simulink model "BLDC"  (R2014b)
settings: Solver=ode45  StartTime=0.0  StopTime=.3  MaxStep=.0001  RelTol=1e-3
values from neighbouring files (symbols this model uses):
  A = [-r/l,0,0,0 ... (first row only)    [motorParams.m]
  B = [2/(3*l),1/(3*l),0 ... (first row only)    [motorParams.m]
  C = [1,0,0,0 ... (first row only)    [motorParams.m]
  c0 = .001    (= 0.001)    [motorParams.m]
  D = [0,0,0 ... (first row only)    [motorParams.m]
  encoderResolution = 12    [motorParams.m]
  encoderSampleTime = .001    (= 0.001)    [motorParams.m]
  ke = 1/(285*2*pi/60)    (= 0.0335063038088)    [motorParams.m]
  kt = 33.5e-3    (= 0.0335)    [motorParams.m]
  p = poles    (= 16)    [motorParams.m]

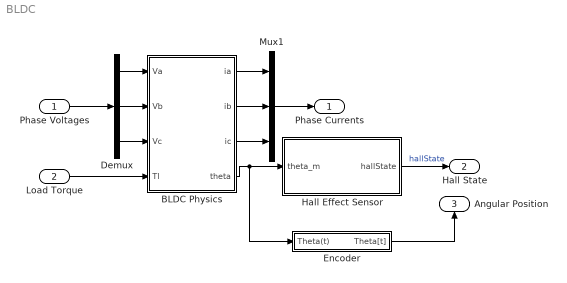
== system BLDC ==
  Phase Voltages : Inport  OutDataTypeStr=double  PortDimensions=3  SampleTime=0
  Load Torque : Inport  Port=2  OutDataTypeStr=double  PortDimensions=1  SampleTime=[0,0]
  BLDC Physics : Subsystem
  Demux : Demux  Outputs=3
  Encoder : Subsystem
  Hall Effect Sensor : MATLAB Function  TreatAsAtomicUnit=on
  Mux1 : Mux  Inputs=3
  Phase Currents : Outport  OutDataTypeStr=double  PortDimensions=3  SampleTime=0
  Hall State : Outport  Port=2  OutDataTypeStr=double  PortDimensions=[1 3]  SampleTime=0
  Angular Position : Outport  Port=3  OutDataTypeStr=double  PortDimensions=1  SampleTime=[0.001,0]
  wires:
  Hall Effect Sensor/1(hallState) -> Hall State/1  "hallState"
  Load Torque/1 -> BLDC Physics/4(Tl)
  BLDC Physics/4(theta) -> Hall Effect Sensor/1(theta_m), Encoder/1(Theta(t))
  Mux1/1 -> Phase Currents/1
  BLDC Physics/3(ic) -> Mux1/3
  BLDC Physics/2(ib) -> Mux1/2
  BLDC Physics/1(ia) -> Mux1/1
  Demux/3 -> BLDC Physics/3(Vc)
  Phase Voltages/1 -> Demux/1
  Demux/1 -> BLDC Physics/1(Va)
  Demux/2 -> BLDC Physics/2(Vb)
  Encoder/1("Theta[t] ") -> Angular Position/1

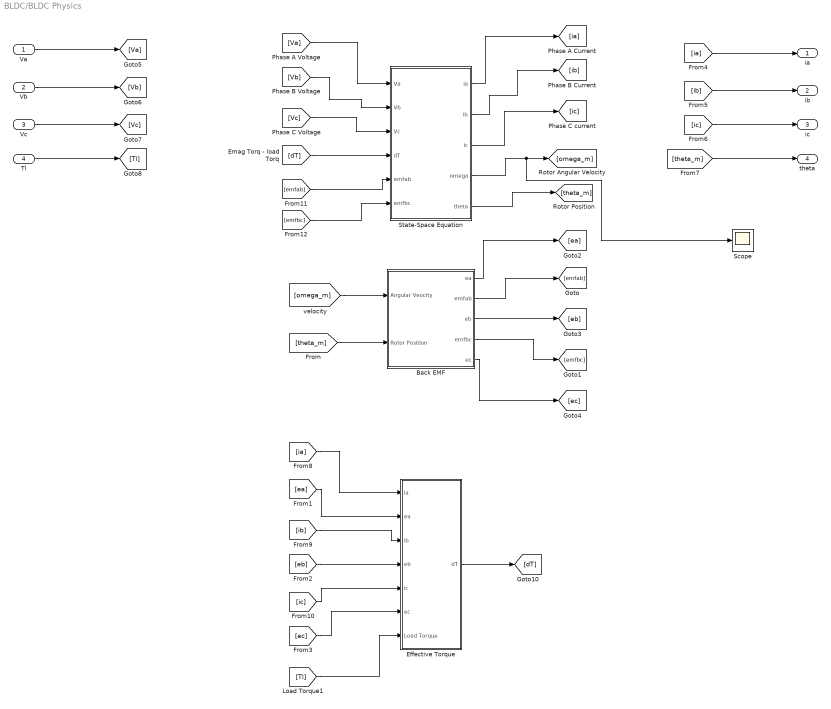
== system BLDC/BLDC Physics ==
  Va : Inport
  Vb : Inport  Port=2
  Vc : Inport  Port=3
  Tl : Inport  Port=4
  Back EMF : Subsystem
  Effective Torque : Subsystem
  Scope : Scope
  State-Space Equation : Subsystem
  ia : Outport
  ib : Outport  Port=2
  ic : Outport  Port=3
  theta : Outport  Port=4
  wires:
  [emfbc] -> State-Space Equation/6(emfbc)
  [emfab] -> State-Space Equation/5(emfab)
  Back EMF/4(emfbc) -> [emfbc]
  Vb/1 -> [Vb]
  Va/1 -> [Va]
  [theta_m] -> Back EMF/2(Rotor Position)
  Back EMF/1(ea) -> [ea]
  Tl/1 -> [Tl]
  [ia] -> ia/1
  [theta_m] -> theta/1
  Back EMF/3(eb) -> [eb]
  [ic] -> ic/1
  Vc/1 -> [Vc]
  [ib] -> ib/1
  Back EMF/5(ec) -> [ec]
  [omega_m] -> Back EMF/1(Angular Veocity)
  Back EMF/2(emfab) -> [emfab]
  [eb] -> Effective Torque/4(eb)
  [Tl] -> Effective Torque/7(Load Torque)
  [ic] -> Effective Torque/5(ic)
  [ea] -> Effective Torque/2(ea)
  [ia] -> Effective Torque/1(ia)
  [ec] -> Effective Torque/6(ec)
  [ib] -> Effective Torque/3(ib)
  Effective Torque/1(dT) -> [dT]
  [Vc] -> State-Space Equation/3(Vc)
  State-Space Equation/3(ic) -> [ic]
  State-Space Equation/4(omega) -> [omega_m], Scope/1
  [Vb] -> State-Space Equation/2(Vb)
  [dT] -> State-Space Equation/4(dT)
  State-Space Equation/2(ib) -> [ib]
  State-Space Equation/5(theta) -> [theta_m]
  [Va] -> State-Space Equation/1(Va)
  State-Space Equation/1(ia) -> [ia]

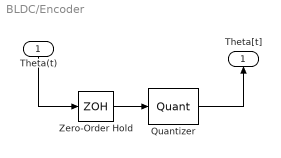
== system BLDC/Encoder ==
  Theta(t) : Inport
  Quantizer : Quantizer  QuantizationInterval=2*pi/(2^encoderResolution)
  Zero-Order Hold : ZeroOrderHold  SampleTime=encoderSampleTime
  "Theta[t] " : Outport
  wires:
  Zero-Order Hold/1 -> Quantizer/1
  Theta(t)/1 -> Zero-Order Hold/1
  Quantizer/1 -> "Theta[t] "/1

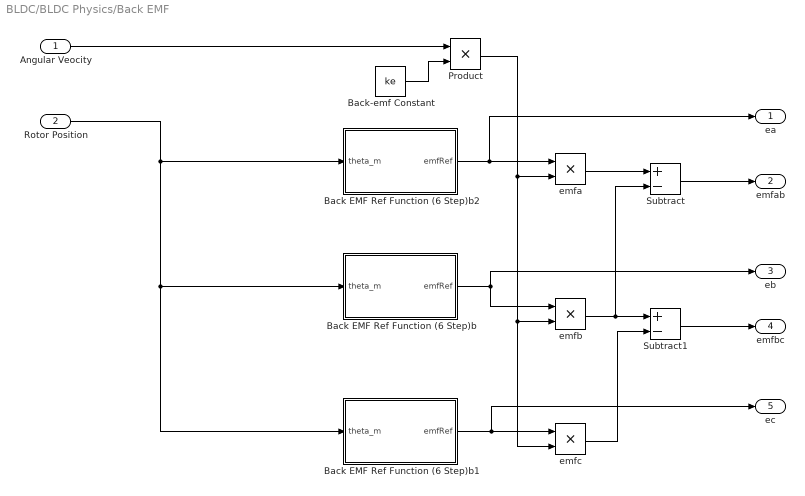
== system BLDC/BLDC Physics/Back EMF ==
  Angular Veocity : Inport
  Rotor Position : Inport  Port=2
  Back EMF Ref Function (6 Step)b : MATLAB Function  TreatAsAtomicUnit=on  mask{offset=-2*pi/3, p=p}
      mask prompts: offset "Phase shift"; p "Number of poles"
  Back EMF Ref Function (6 Step)b1 : MATLAB Function  TreatAsAtomicUnit=on  mask{offset=2*pi/3, p=p}
      mask prompts: offset "Phase shift"; p "Number of poles"
  Back EMF Ref Function (6 Step)b2 : MATLAB Function  TreatAsAtomicUnit=on  mask{offset=0, p=p}
      mask prompts: offset "Phase shift"; p "Number of poles"
  Back-emf Constant : Constant  Value=ke
  Product : Product
  Subtract : Sum  Inputs=+-
  Subtract1 : Sum  Inputs=+-
  emfa : Product
  emfb : Product
  emfc : Product
  ea : Outport
  emfab : Outport  Port=2
  eb : Outport  Port=3
  emfbc : Outport  Port=4
  ec : Outport  Port=5
  wires:
  Subtract1/1 -> emfbc/1
  Subtract/1 -> emfab/1
  emfa/1 -> Subtract/1
  Angular Veocity/1 -> Product/1
  Back EMF Ref Function (6 Step)b1/1(emfRef) -> emfc/1, ec/1
  Back EMF Ref Function (6 Step)b/1(emfRef) -> emfb/1, eb/1
  emfb/1 -> Subtract1/1, Subtract/2
  Product/1 -> emfb/2, emfc/2, emfa/2
  Back-emf Constant/1 -> Product/2
  emfc/1 -> Subtract1/2
  Back EMF Ref Function (6 Step)b2/1(emfRef) -> emfa/1, ea/1
  Rotor Position/1 -> Back EMF Ref Function (6 Step)b/1(theta_m), Back EMF Ref Function (6 Step)b1/1(theta_m), Back EMF Ref Function (6 Step)b2/1(theta_m)

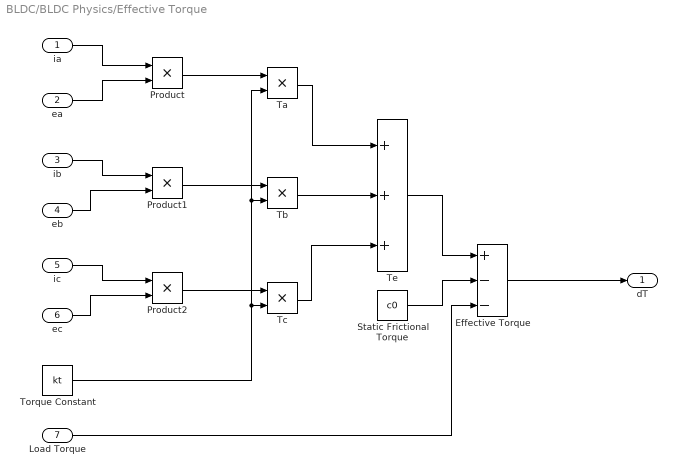
== system BLDC/BLDC Physics/Effective Torque ==
  ia : Inport
  ea : Inport  Port=2
  ib : Inport  Port=3
  eb : Inport  Port=4
  ic : Inport  Port=5
  ec : Inport  Port=6
  Load Torque : Inport  Port=7
  Effective Torque : Sum  Inputs=+--
  Product : Product
  Product1 : Product
  Product2 : Product
  Static Frictional Torque : Constant  Value=c0
  Ta : Product  Inputs=**
  Tb : Product  Inputs=**
  Tc : Product  Inputs=**
  Te : Sum  Inputs=+++
  Torque Constant : Constant  Value=kt
  dT : Outport
  wires:
  Te/1 -> Effective Torque/1
  Product2/1 -> Tc/1
  Product1/1 -> Tb/1
  Product/1 -> Ta/1
  Torque Constant/1 -> Ta/2, Tb/2, Tc/2
  Effective Torque/1 -> dT/1
  ia/1 -> Product/1
  ic/1 -> Product2/1
  ea/1 -> Product/2
  ib/1 -> Product1/1
  eb/1 -> Product1/2
  ec/1 -> Product2/2
  Tb/1 -> Te/2
  Ta/1 -> Te/1
  Tc/1 -> Te/3
  Load Torque/1 -> Effective Torque/3
  Static Frictional Torque/1 -> Effective Torque/2

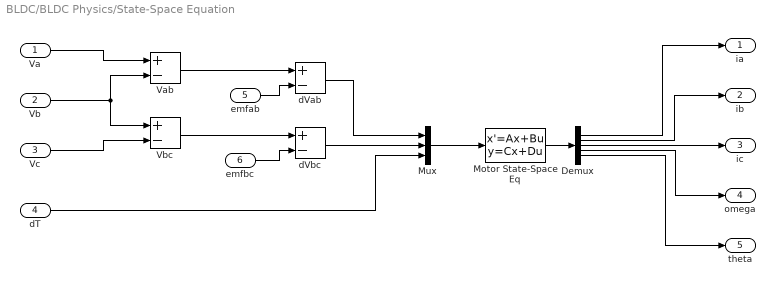
== system BLDC/BLDC Physics/State-Space Equation ==
  Va : Inport
  Vb : Inport  Port=2
  Vc : Inport  Port=3
  dT : Inport  Port=4
  emfab : Inport  Port=5
  emfbc : Inport  Port=6
  Demux : Demux  Outputs=5
  Motor State-Space Eq : StateSpace  A=A  B=B  C=C  D=D  X0=0
  Mux : Mux  Inputs=3
  Vab : Sum  Inputs=+-
  Vbc : Sum  Inputs=+-
  dVab : Sum  Inputs=+-
  dVbc : Sum  Inputs=+-
  ia : Outport
  ib : Outport  Port=2
  ic : Outport  Port=3
  omega : Outport  Port=4
  theta : Outport  Port=5
  wires:
  Vc/1 -> Vbc/2
  Vb/1 -> Vbc/1, Vab/2
  Va/1 -> Vab/1
  emfab/1 -> dVab/2
  dVab/1 -> Mux/1
  Vab/1 -> dVab/1
  Vbc/1 -> dVbc/1
  dT/1 -> Mux/3
  Mux/1 -> Motor State-Space Eq/1
  emfbc/1 -> dVbc/2
  Motor State-Space Eq/1 -> Demux/1
  Demux/4 -> omega/1
  Demux/1 -> ia/1
  Demux/3 -> ic/1
  Demux/5 -> theta/1
  Demux/2 -> ib/1
  dVbc/1 -> Mux/2

== matlab function BLDC/BLDC Physics/Back EMF/Back EMF Ref Function (6 Step)b ==
function emfRef = F(theta_m, p, offset)
    theta_e = (p/2).*theta_m + offset;
    theta_e = mod(theta_e, (2*pi));
    if theta_e < 0
        theta_e = 2*pi - theta_e;
    end
    if (theta_e <= 2*pi/3)
        emfRef = 1;
    elseif (theta_e <= pi)
        emfRef = 1-(6/pi)*(theta_e - 2*pi/3);
    elseif (theta_e <= 5*pi/3)
        emfRef = -1;
    else
        emfRef = -1 + (6/pi)*(theta_e - 5*pi/3);
    end

end

== matlab function BLDC/BLDC Physics/Back EMF/Back EMF Ref Function (6 Step)b1 ==
function emfRef = F(theta_m, p, offset)
    theta_e = (p/2).*theta_m + offset;
    theta_e = mod(theta_e, (2*pi));
    if theta_e < 0
        theta_e = 2*pi - theta_e;
    end
    if (theta_e <= 2*pi/3)
        emfRef = 1;
    elseif (theta_e <= pi)
        emfRef = 1-(6/pi)*(theta_e - 2*pi/3);
    elseif (theta_e <= 5*pi/3)
        emfRef = -1;
    else
        emfRef = -1 + (6/pi)*(theta_e - 5*pi/3);
    end

end

== matlab function BLDC/BLDC Physics/Back EMF/Back EMF Ref Function (6 Step)b2 ==
function emfRef = F(theta_m, p, offset)
    theta_e = (p/2).*theta_m + offset;
    theta_e = mod(theta_e, (2*pi));
    if theta_e < 0
        theta_e = 2*pi - theta_e;
    end
    if (theta_e <= 2*pi/3)
        emfRef = 1;
    elseif (theta_e <= pi)
        emfRef = 1-(6/pi)*(theta_e - 2*pi/3);
    elseif (theta_e <= 5*pi/3)
        emfRef = -1;
    else
        emfRef = -1 + (6/pi)*(theta_e - 5*pi/3);
    end

end

== matlab function BLDC/Hall Effect Sensor ==
function hallState = hallEffectSensor(poles,theta_m)
	theta_e = (poles/2).*theta_m;
    theta_e = mod(theta_e, (2*pi));
    if theta_e < 0
        theta_e = 2*pi - theta_e;
    end
    
    if theta_e <= pi/3
        hallState = [1 0 0];
    elseif theta_e <= 2*pi/3
        hallState = [1 1 0];
    elseif theta_e <= pi
        hallState = [0 1 0];
    elseif theta_e <= 4*pi/3
        hallState = [0 1 1];
    elseif theta_e <= 5*pi/3
        hallState = [0 0 1];
    elseif theta_e <= 2*pi
        hallState = [1 0 1];
    else 
        hallState = [0 0 0]; %%Error Code, should never occur in Sim...
    end
